simulink model "apinv"  (Simulink 3.00)
settings: Solver=ode45  SolverMode=SingleTasking  StartTime=0.0  StopTime=100  MaxStep=0.10  RelTol=1e-4  AbsTol=1e-4
settings Model: TimeSaveName=t  SaveOutput=off

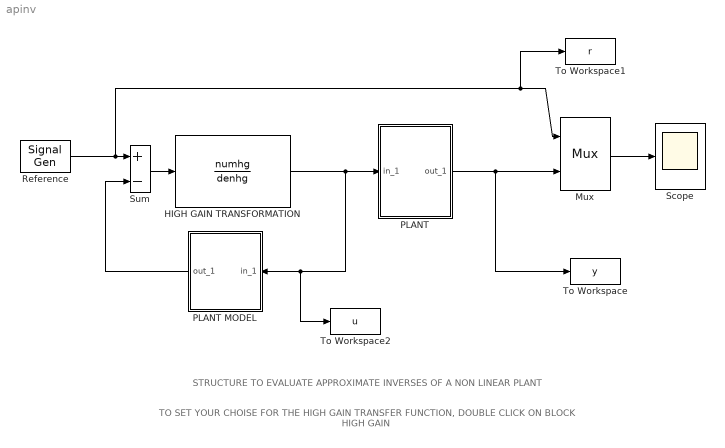
== system apinv ==
  note: STRUCTURE TO EVALUATE APPROXIMATE INVERSES OF A NON LINEAR PLANT
  note: TO SET YOUR CHOISE FOR THE HIGH GAIN TRANSFER FUNCTION,
      |  DOUBLE CLICK ON BLOCK HIGH GAIN
  HIGH GAIN TRANSFORMATION : TransferFcn  Numerator=numhg  Denominator=denhg  mask(HIGH GAIN TRANSFORMATION){@1=[0.5 1.6 1.28], @2=[1 2 0]}
      mask prompts: @1 "numerator:"; @2 "denominator:"
      mask help: HIGH GAIN LINEAR TRANSFORMATION
      mask init:
      | numhg=@1;denhg=@2;
      mask Display: disp('HIGH GAIN ')
  Mux : Mux  Inputs=2
      settings: DisplayOption=none
  PLANT : Subsystem
      mask Type: Plant
      mask Display: disp('Plant')
  PLANT MODEL : Subsystem  Orientation=left
      mask Type: Model
      mask Display: disp('Model')
  Reference : SignalGenerator  WaveForm=sine  Amplitude=1.000000  Frequency=0.250000  Units=rad/sec
  Scope : Scope
      settings: TickLabels=on  TimeRange=100.000000  YMin=-2  YMax=2  SaveToWorkspace=off  SaveName=ScopeData  DataFormat=Matrix
  Sum : Sum  Inputs=+-  SaturateOnIntegerOverflow=on
  To Workspace : ToWorkspace  VariableName=y  SampleTime=0  SaveFormat=Matrix
      settings: Buffer=10000
  To Workspace1 : ToWorkspace  VariableName=r  SampleTime=0  SaveFormat=Matrix
      settings: Buffer=10000
  To Workspace2 : ToWorkspace  VariableName=u  SampleTime=0  SaveFormat=Matrix
      settings: Buffer=10000
  wires:
  Sum/1 -> HIGH GAIN TRANSFORMATION/1
  Mux/1 -> Scope/1
  PLANT MODEL/1(out_1) -> Sum/2
  Reference/1 -> Sum/1, Mux/1, To Workspace1/1
  PLANT/1(out_1) -> Mux/2, To Workspace/1
  HIGH GAIN TRANSFORMATION/1 -> PLANT/1(in_1), PLANT MODEL/1(in_1), To Workspace2/1

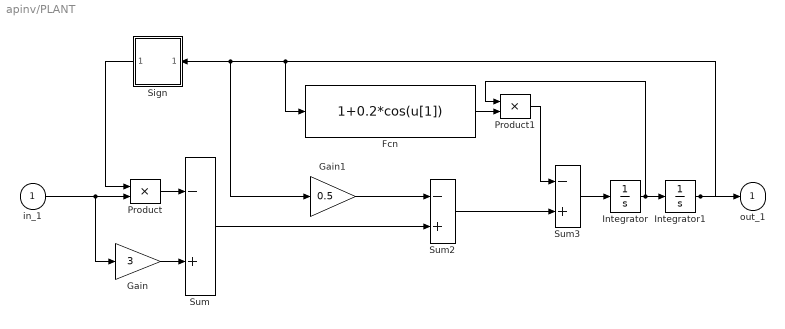
== system apinv/PLANT ==
  in_1 : Inport  Port=1  PortWidth=-1  SampleTime=-1  DataType=auto
      settings: SignalType=auto
  Fcn : Fcn  Expr=1+0.2*cos(u[1])
  Gain : Gain  Gain=3  SaturateOnIntegerOverflow=on
  Gain1 : Gain  Gain=0.5  SaturateOnIntegerOverflow=on
  Integrator : Integrator  ExternalReset=none  InitialConditionSource=internal  InitialCondition=0  LimitOutput=off  UpperSaturationLimit=inf  LowerSaturationLimit=-inf  ShowSaturationPort=off  ShowStatePort=off  AbsoluteTolerance=auto
  Integrator1 : Integrator  ExternalReset=none  InitialConditionSource=internal  InitialCondition=0  LimitOutput=off  UpperSaturationLimit=inf  LowerSaturationLimit=-inf  ShowSaturationPort=off  ShowStatePort=off  AbsoluteTolerance=auto
  Product : Product  Inputs=2  SaturateOnIntegerOverflow=on
  Product1 : Product  Inputs=2  SaturateOnIntegerOverflow=on
  Sign : Subsystem  Orientation=left
      mask Type: Sign
      mask Description: y = sign(x)
      mask Help: Sign Function:\n\t\t\ty = 1 if x > 0\n\t\t\ty = 0 if x = 0\n\t\t\ty = -1 if x < 0
      mask Display: plot(-50,-50,50,50,[-50,50],[0,0],[0,0],[-50,50],[-40,0],[-30,-30],[0,40],[30,30])
  Sum : Sum  Inputs=-+  SaturateOnIntegerOverflow=on
  Sum2 : Sum  Inputs=-+  SaturateOnIntegerOverflow=on
  Sum3 : Sum  Inputs=-+  SaturateOnIntegerOverflow=on
  out_1 : Outport  Port=1  InitialOutput=0
  wires:
  Integrator/1 -> Integrator1/1, Product1/1
  Sum3/1 -> Integrator/1
  Sum2/1 -> Sum3/2
  Fcn/1 -> Product1/2
  Gain1/1 -> Sum2/1
  Sign/1(out_1) -> Product/1
  Sum/1 -> Sum2/2
  in_1/1 -> Product/2, Gain/1
  Gain/1 -> Sum/2
  Product/1 -> Sum/1
  Integrator1/1 -> Fcn/1, Sign/1(in_1), Gain1/1, out_1/1
  Product1/1 -> Sum3/1

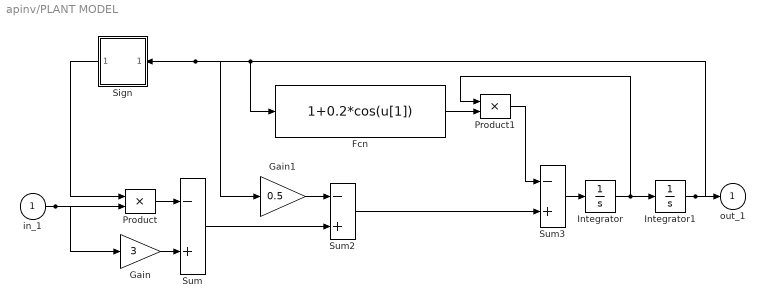
== system apinv/PLANT MODEL ==
  in_1 : Inport  Port=1  PortWidth=-1  SampleTime=-1  DataType=auto
      settings: SignalType=auto
  Fcn : Fcn  Expr=1+0.2*cos(u[1])
  Gain : Gain  Gain=3  SaturateOnIntegerOverflow=on
  Gain1 : Gain  Gain=0.5  SaturateOnIntegerOverflow=on
  Integrator : Integrator  ExternalReset=none  InitialConditionSource=internal  InitialCondition=0  LimitOutput=off  UpperSaturationLimit=inf  LowerSaturationLimit=-inf  ShowSaturationPort=off  ShowStatePort=off  AbsoluteTolerance=auto
  Integrator1 : Integrator  ExternalReset=none  InitialConditionSource=internal  InitialCondition=0  LimitOutput=off  UpperSaturationLimit=inf  LowerSaturationLimit=-inf  ShowSaturationPort=off  ShowStatePort=off  AbsoluteTolerance=auto
  Product : Product  Inputs=2  SaturateOnIntegerOverflow=on
  Product1 : Product  Inputs=2  SaturateOnIntegerOverflow=on
  Sign : Subsystem  Orientation=left
      mask Type: Sign
      mask Description: y = sign(x)
      mask Help: Sign Function:\n\t\t\ty = 1 if x > 0\n\t\t\ty = 0 if x = 0\n\t\t\ty = -1 if x < 0
      mask Display: plot(-50,-50,50,50,[-50,50],[0,0],[0,0],[-50,50],[-40,0],[-30,-30],[0,40],[30,30])
  Sum : Sum  Inputs=-+  SaturateOnIntegerOverflow=on
  Sum2 : Sum  Inputs=-+  SaturateOnIntegerOverflow=on
  Sum3 : Sum  Inputs=-+  SaturateOnIntegerOverflow=on
  out_1 : Outport  Port=1  InitialOutput=0
  wires:
  Product1/1 -> Sum3/1
  Integrator/1 -> Integrator1/1, Product1/1
  Sum3/1 -> Integrator/1
  Sum2/1 -> Sum3/2
  Fcn/1 -> Product1/2
  Gain1/1 -> Sum2/1
  Sign/1(out_1) -> Product/1
  Sum/1 -> Sum2/2
  Gain/1 -> Sum/2
  Product/1 -> Sum/1
  Integrator1/1 -> Fcn/1, Sign/1(in_1), Gain1/1, out_1/1
  in_1/1 -> Product/2, Gain/1

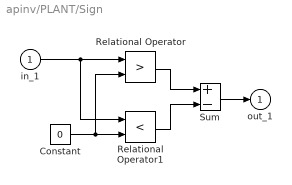
== system apinv/PLANT/Sign ==
  in_1 : Inport  Port=1  PortWidth=-1  SampleTime=-1  DataType=auto
      settings: SignalType=auto
  Constant : Constant  Value=0
  Relational Operator : RelationalOperator  Operator=>
  Relational Operator1 : RelationalOperator  Operator=<
  Sum : Sum  Inputs=+-  SaturateOnIntegerOverflow=on
  out_1 : Outport  Port=1  InitialOutput=0
  wires:
  in_1/1 -> Relational Operator/1, Relational Operator1/1
  Constant/1 -> Relational Operator1/2, Relational Operator/2
  Relational Operator1/1 -> Sum/2
  Relational Operator/1 -> Sum/1
  Sum/1 -> out_1/1

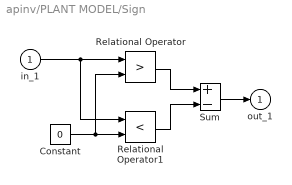
== system apinv/PLANT MODEL/Sign ==
  in_1 : Inport  Port=1  PortWidth=-1  SampleTime=-1  DataType=auto
      settings: SignalType=auto
  Constant : Constant  Value=0
  Relational Operator : RelationalOperator  Operator=>
  Relational Operator1 : RelationalOperator  Operator=<
  Sum : Sum  Inputs=+-  SaturateOnIntegerOverflow=on
  out_1 : Outport  Port=1  InitialOutput=0
  wires:
  in_1/1 -> Relational Operator/1, Relational Operator1/1
  Constant/1 -> Relational Operator1/2, Relational Operator/2
  Relational Operator1/1 -> Sum/2
  Relational Operator/1 -> Sum/1
  Sum/1 -> out_1/1
